simulink model "util_common_hrn"  (R2014b)
settings: Solver=FixedStepDiscrete  StartTime=0.0  StopTime=1  FixedStep=.1  MaxStep=.1  RelTol=1e-3
values from neighbouring files (symbols this model uses):
  noise_generator_bias = [10 10 10]    [util_common_test.m]
  noise_generator_sample_time = 0.1    [util_common_test.m]
  noise_generator_seed = [50 51 49]    [util_common_test.m]
  noise_generator_std_deviation = [5 5 5]    [util_common_test.m]
  ramp_Initial_Output = 0    [util_common_test.m]
  ramp_Slope = 1    [util_common_test.m]
libraries: util_common_lib x15
settings Model: RequirementInfo={'other' 'util_common_req.html' '' 'true' 'Requirements for Common Math and Signal libraries' '' } %GIDa_df6e5ca7_455d_4fd0_87bf_28496eb10a22  ExtModeAutoUpdateStatusClock=off  Creator=hcannon  LastModifiedBy=mstewart
settings DataIOCC: SignalLoggingSaveFormat=ModelDataLogs
settings OptimizationCC: ExpressionDepthLimit=2147483647  InitFltsAndDblsToZero=on
settings DebuggingCC: UnderspecifiedInitializationDetection=Classic  MergeDetectMultiDrivingBlocksExec=none  FcnCallInpInsideContextMsg=UseLocalSettings  StateNameClashWarn=warning  StrictBusMsg=Warning
settings GRTTargetCC: CombineOutputUpdateFcns=off  GRTInterface=on

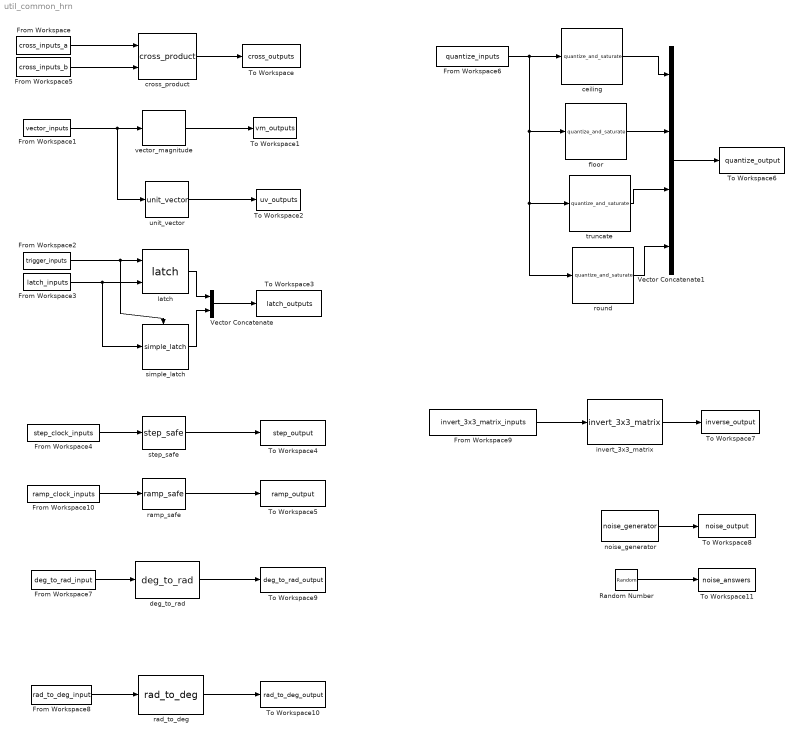
== system util_common_hrn ==
  From Workspace : FromWorkspace  VariableName=cross_inputs_a  SampleTime=0
  From Workspace1 : FromWorkspace  VariableName=vector_inputs  SampleTime=0
  From Workspace10 : FromWorkspace  VariableName=ramp_clock_inputs  SampleTime=0
  From Workspace2 : FromWorkspace  VariableName=trigger_inputs  SampleTime=0  Interpolate=off  OutputAfterFinalValue=Setting to zero
  From Workspace3 : FromWorkspace  VariableName=latch_inputs  SampleTime=0
  From Workspace4 : FromWorkspace  VariableName=step_clock_inputs  SampleTime=0
  From Workspace5 : FromWorkspace  VariableName=cross_inputs_b  SampleTime=0
  From Workspace6 : FromWorkspace  VariableName=quantize_inputs  SampleTime=0
  From Workspace7 : FromWorkspace  VariableName=deg_to_rad_input  SampleTime=0
  From Workspace8 : FromWorkspace  VariableName=rad_to_deg_input  SampleTime=0
  From Workspace9 : FromWorkspace  VariableName=invert_3x3_matrix_inputs  SampleTime=0
  Random Number : RandomNumber  Mean=noise_generator_bias  Variance=noise_generator_std_deviation.^2  Seed=noise_generator_seed  SampleTime=noise_generator_sample_time
  To Workspace : ToWorkspace  VariableName=cross_outputs  SampleTime=-1
  To Workspace1 : ToWorkspace  VariableName=vm_outputs  SampleTime=-1
  To Workspace10 : ToWorkspace  VariableName=rad_to_deg_output  SampleTime=-1
  To Workspace11 : ToWorkspace  VariableName=noise_answers  SampleTime=-1
  To Workspace2 : ToWorkspace  VariableName=uv_outputs  SampleTime=-1
  To Workspace3 : ToWorkspace  VariableName=latch_outputs  SaveFormat=Structure With Time  SampleTime=-1
  To Workspace4 : ToWorkspace  VariableName=step_output  SampleTime=-1
  To Workspace5 : ToWorkspace  VariableName=ramp_output  SampleTime=-1
  To Workspace6 : ToWorkspace  VariableName=quantize_output  SampleTime=-1
  To Workspace7 : ToWorkspace  VariableName=inverse_output  SampleTime=-1
  To Workspace8 : ToWorkspace  VariableName=noise_output  SampleTime=-1
  To Workspace9 : ToWorkspace  VariableName=deg_to_rad_output  SampleTime=-1
  Vector Concatenate : Concatenate
  Vector Concatenate1 : Concatenate  NumInputs=4
  ceiling : util_common_lib/quantize_and_saturate  RES=quantize_and_saturate_Resolution  OPER=ceil  out_min=quantize_and_saturate_Output_Minimum  out_max=quantize_and_saturate_Output_Maximum
  cross_product : util_common_lib/cross_product  SystemSampleTime=-1
  deg_to_rad : util_common_lib/deg_to_rad  SystemSampleTime=-1
  floor : util_common_lib/quantize_and_saturate  RES=quantize_and_saturate_Resolution  OPER=floor  out_min=quantize_and_saturate_Output_Minimum  out_max=quantize_and_saturate_Output_Maximum
  invert_3x3_matrix : util_common_lib/invert_3x3_matrix  SystemSampleTime=-1
  latch : util_common_lib/latch  Initial_Latch=latch_Initial_Output_Value
  noise_generator : util_common_lib/noise_generator  std_dev=noise_generator_std_deviation  bias=noise_generator_bias  seed=noise_generator_seed  on=noise_generator_on_flag  sample_time=noise_generator_sample_time
  rad_to_deg : util_common_lib/rad_to_deg  SystemSampleTime=-1
  ramp_safe : util_common_lib/ramp_safe  slope=ramp_Slope  start=ramp_Start_Time  X0=ramp_Initial_Output
  round : util_common_lib/quantize_and_saturate  RES=quantize_and_saturate_Resolution  OPER=round  out_min=quantize_and_saturate_Output_Minimum  out_max=quantize_and_saturate_Output_Maximum
  simple_latch : util_common_lib/simple_latch  SystemSampleTime=-1
  step_safe : util_common_lib/step_safe  step_time=step_Step_Time  initial_value=step_Initial_Value  final_value=step_Final_Value
  truncate : util_common_lib/quantize_and_saturate  RES=quantize_and_saturate_Resolution  OPER=truncate  out_min=quantize_and_saturate_Output_Minimum  out_max=quantize_and_saturate_Output_Maximum
  unit_vector : util_common_lib/unit_vector  SystemSampleTime=-1
  vector_magnitude : util_common_lib/vector_magnitude  SystemSampleTime=-1
  wires:
  From Workspace/1 -> cross_product/1
  cross_product/1 -> To Workspace/1
  From Workspace1/1 -> vector_magnitude/1, unit_vector/1
  vector_magnitude/1 -> To Workspace1/1
  unit_vector/1 -> To Workspace2/1
  From Workspace5/1 -> cross_product/2
  From Workspace3/1 -> latch/2, simple_latch/1
  From Workspace2/1 -> latch/1, simple_latch/Trigger
  latch/1 -> Vector Concatenate/1
  simple_latch/1 -> Vector Concatenate/2
  Vector Concatenate/1 -> To Workspace3/1
  step_safe/1 -> To Workspace4/1
  ramp_safe/1 -> To Workspace5/1
  From Workspace6/1 -> ceiling/1, floor/1, truncate/1, round/1
  ceiling/1 -> Vector Concatenate1/1
  floor/1 -> Vector Concatenate1/2
  truncate/1 -> Vector Concatenate1/3
  round/1 -> Vector Concatenate1/4
  Vector Concatenate1/1 -> To Workspace6/1
  invert_3x3_matrix/1 -> To Workspace7/1
  noise_generator/1 -> To Workspace8/1
  From Workspace7/1 -> deg_to_rad/1
  From Workspace8/1 -> rad_to_deg/1
  deg_to_rad/1 -> To Workspace9/1
  rad_to_deg/1 -> To Workspace10/1
  From Workspace9/1 -> invert_3x3_matrix/1
  Random Number/1 -> To Workspace11/1
  From Workspace4/1 -> step_safe/1
  From Workspace10/1 -> ramp_safe/1
